simulink model "ControlDesignHarness"  (R2017b)
settings: configuration reference "ControlDesignConfigSet" (kept outside this file)
settings Model: Creator=eh6qym  LastModifiedBy=eh6qym
settings ConfigSetRef: SourceLocation=Base Workspace

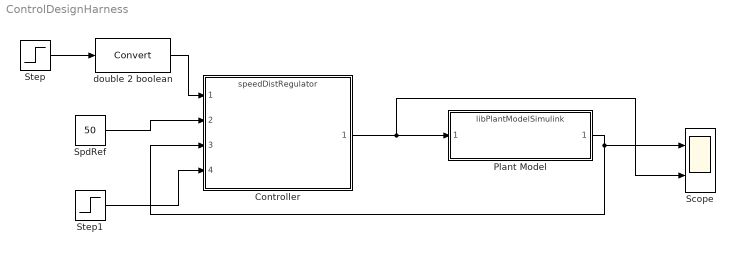
== system ControlDesignHarness ==
  Controller : ModelReference  ModelNameDialog=speedDistRegulator.slx  SimulationMode=Normal  ModelReferenceVersion=1.36
  Plant Model : ModelReference  ModelNameDialog=libPlantModelSimulink.mdl  SimulationMode=Normal  ModelReferenceVersion=1.22
  Scope : Scope  NumInputPorts=2
  SpdRef : Constant  Value=50
  Step : Step  SampleTime=0
  Step1 : Step  Time=70  Before=50  After=20  SampleTime=0
  double 2 boolean : DataTypeConversion
  wires:
  Controller/1 -> Scope/2, Plant Model/1
  SpdRef/1 -> Controller/2
  Plant Model/1 -> Scope/1, Controller/3
  Step/1 -> double 2 boolean/1
  double 2 boolean/1 -> Controller/1
  Step1/1 -> Controller/4
